simulink model "calibration_model_v2_phase_pid"  (R2015b)
settings: Solver=FixedStepDiscrete  StartTime=0.0  StopTime=inf  FixedStep=.001  RelTol=1e-3
libraries: xpcethercatlib x10, slrtlib x5, simulink x1, dspfdesign x1
settings Model: xpc_rtwmakecfg_data=_xpcethercatlib_  SimulationMode=external  Creator=rtheyyun  LastModifiedBy=tech
settings SolverCC: EnableConcurrentExecution=on  ConcurrentTasks=on
settings DataIOCC: SaveFinalState=on  SaveFormat=StructureWithTime  SignalLoggingSaveFormat=ModelDataLogs  InspectSignalLogs=on
settings OptimizationCC: BlockReduction=off  OptimizeBlockIOStorage=off  BufferReuse=off  GlobalBufferReuse=off  ExpressionFolding=off  ExpressionDepthLimit=2147483647  LocalBlockOutputs=off
settings DebuggingCC: ReadBeforeWriteMsg=DisableAll  WriteAfterWriteMsg=DisableAll  WriteAfterReadMsg=DisableAll  UnderspecifiedInitializationDetection=Classic  MergeDetectMultiDrivingBlocksExec=none  SolverPrmCheckMsg=warning  InheritedTsInSrcMsg=none  FcnCallInpInsideContextMsg=UseLocalSettings  StateNameClashWarn=warning
settings HardwareCC: ProdBitPerPointer=32  ProdLargestAtomicFloat=None  ProdWordSize=32  ProdLongLongMode=on  ProdHWDeviceType=Generic->32-bit x86 compatible
settings RTWCC: SystemTargetFile=slrt.tlc  TemplateMakefile=slrt_default_tmf  Description=Simulink Real-Time  RTWVerbose=off  RTWCompilerOptimization=on
settings SimulinkRealTimeCC: GeneratePreprocessorConditionals=Disable all  xPCisModelTimeout=off  xPCModelTimeoutSecs=20  xPCConcurrentTasks=on
settings ConfigComp: CovModelRefEnable=Off  CovSFcnEnable=off

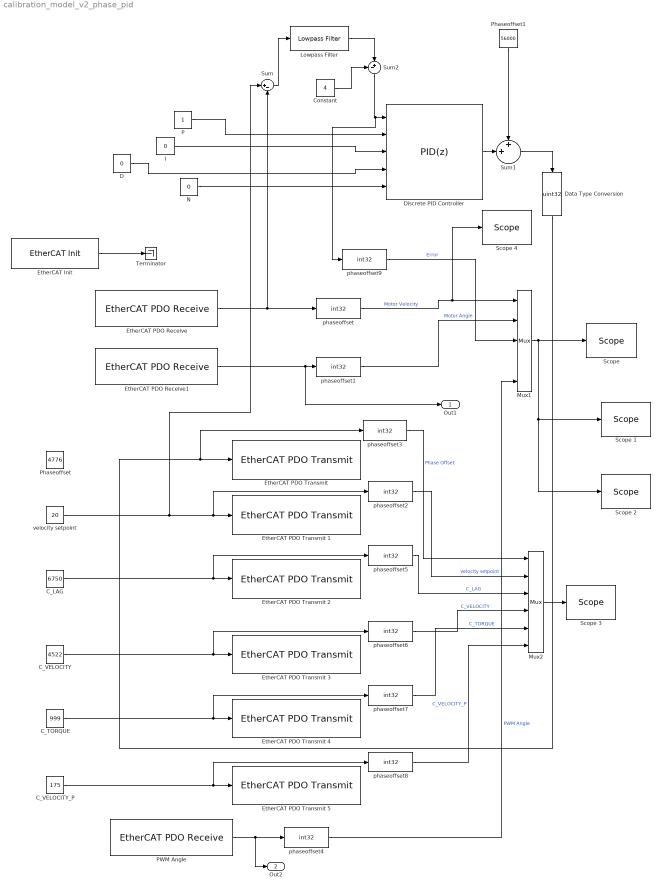
== system calibration_model_v2_phase_pid ==
  C_LAG : Constant  Value=6750  OutDataTypeStr=uint32
  C_TORQUE : Constant  Value=999  OutDataTypeStr=uint32
  C_VELOCITY : Constant  Value=4522  OutDataTypeStr=uint32
  C_VELOCITY_P : Constant  Value=175  OutDataTypeStr=uint32
  Constant : Constant  Value=4
  D : Constant  Value=0
  Data Type Conversion : DataTypeConversion  OutDataTypeStr=uint32
  Discrete PID Controller : simulink/Continuous/PID Controller  Controller=PID  TimeDomain=Discrete-time  SampleTime=-1  IntegratorMethod=Forward Euler  FilterMethod=Forward Euler  Form=Parallel  UseFilter=on  ControllerParametersSource=external  P=1  I=1  D=0  N=100  InitialConditionSource=internal  InitialConditionForIntegrator=0  InitialConditionForFilter=0  ExternalReset=none  LimitOutput=on  UpperSaturationLimit=25536  LowerSaturationLimit=-40000  LinearizeAsGain=off  AntiWindupMode=none  Kb=1  TrackingMode=off  Kt=1  PParamMin=[]  PParamMax=[]  IParamMin=[]  IParamMax=[]  DParamMin=[]  DParamMax=[]  NParamMin=[]  NParamMax=[]  KbParamMin=[]  KbParamMax=[]  KtParamMin=[]  KtParamMax=[]  POutMin=[]  POutMax=[]  IOutMin=[]  IOutMax=[]  DOutMin=[]  DOutMax=[]  NOutMin=[]  NOutMax=[]  KbOutMin=[]  KbOutMax=[]  KtOutMin=[]  KtOutMax=[]  IntegratorOutMin=[]  IntegratorOutMax=[]  FilterOutMin=[]  FilterOutMax=[]  SumOutMin=[]  SumOutMax=[]  SumI1OutMin=[]  SumI1OutMax=[]  SumI2OutMin=[]  SumI2OutMax=[]  SumI3OutMin=[]  SumI3OutMax=[]  SumDOutMin=[]  SumDOutMax=[]  SaturationOutMin=[]  SaturationOutMax=[]  IntegratorContinuousStateAttributes=''  IntegratorStateMustResolveToSignalObject=off  IntegratorRTWStateStorageClass=Auto  FilterContinuousStateAttributes=''  FilterStateMustResolveToSignalObject=off  FilterRTWStateStorageClass=Auto  DifferentiatorICPrevScaledInput=0  DifferentiatorOutMin=[]  DifferentiatorOutMax=[]
  "EtherCAT Init " : xpcethercatlib/EtherCAT Init   Priority=0  config_file=C:\Software\Simulink Realtime\EtherCAT Config files\single_slave_v1.2.xml  device_id=0  pci_bus=2  pci_slot=0  dctuning=2  enaDebug=off  enaDC=off  errLink=on  masterDbg=on  stateChgDbg=on  baseClock=off  masterCfg=on  logFile='c:\dbglog.txt'  sample_time=0.001000
  EtherCAT PDO Receive : xpcethercatlib/EtherCAT PDO Receive  Priority=2  sig_name=Box 1 (FB1111 SPI-Slave).Inputs.motorVelocity  sig_offset=256  sig_type=int16  type_size=16  sig_dim=1  device_id=0  sample_time=0.001000
  EtherCAT PDO Receive1 : xpcethercatlib/EtherCAT PDO Receive  Priority=2  sig_name=Box 1 (FB1111 SPI-Slave).Inputs.motorAngle  sig_offset=240  sig_type=uint16  type_size=16  sig_dim=1  device_id=0  sample_time=0.001000
  "EtherCAT PDO Transmit " : xpcethercatlib/EtherCAT PDO Transmit   Priority=3  sig_name=Box 1 (FB1111 SPI-Slave).Outputs.jointSetpoint  sig_offset=208  sig_type=uint32  type_size=32  sig_dim=1  device_id=0  sample_time=0.001000
  EtherCAT PDO Transmit 1 : xpcethercatlib/EtherCAT PDO Transmit   Priority=3  sig_name=Box 1 (FB1111 SPI-Slave).Outputs.data0  sig_offset=240  sig_type=uint32  type_size=32  sig_dim=1  device_id=0  sample_time=0.001000
  EtherCAT PDO Transmit 2 : xpcethercatlib/EtherCAT PDO Transmit   Priority=3  sig_name=Box 1 (FB1111 SPI-Slave).Outputs.data1  sig_offset=272  sig_type=uint32  type_size=32  sig_dim=1  device_id=0  sample_time=0.001000
  EtherCAT PDO Transmit 3 : xpcethercatlib/EtherCAT PDO Transmit   Priority=3  sig_name=Box 1 (FB1111 SPI-Slave).Outputs.data2  sig_offset=304  sig_type=uint32  type_size=32  sig_dim=1  device_id=0  sample_time=0.001000
  EtherCAT PDO Transmit 4 : xpcethercatlib/EtherCAT PDO Transmit   Priority=3  sig_name=Box 1 (FB1111 SPI-Slave).Outputs.data3  sig_offset=336  sig_type=uint32  type_size=32  sig_dim=1  device_id=0  sample_time=0.001000
  EtherCAT PDO Transmit 5 : xpcethercatlib/EtherCAT PDO Transmit   Priority=3  sig_name=Box 1 (FB1111 SPI-Slave).Outputs.data4  sig_offset=368  sig_type=uint32  type_size=32  sig_dim=1  device_id=0  sample_time=0.001000
  "I " : Constant  Value=0
  Lowpass Filter : dspfdesign/Lowpass Filter  FilterType=FIR  DesignForMinimumOrder=on  FilterOrder=50  PassbandFrequency=10  StopbandFrequency=20  PassbandRipple=0.1  StopbandAttenuation=80  InheritSampleRate=off  SampleRate=1000  roundingMode=Floor  coeffsDataTypeStr=fixdt(1,16)  SimulateUsing=Interpreted execution
  Mux1 : Mux  Inputs=5
  Mux2 : Mux  Inputs=6
  N : Constant  Value=0
  P : Constant
  PWM Angle : xpcethercatlib/EtherCAT PDO Receive  Priority=2  sig_name=Box 1 (FB1111 SPI-Slave).Inputs.jointAngle  sig_offset=208  sig_type=uint32  type_size=32  sig_dim=1  device_id=0  sample_time=0.001000
  Phaseoffset : Constant  Value=4776  OutDataTypeStr=uint32
  Phaseoffset1 : Constant  Value=56000  OutDataTypeStr=uint32
  "Scope " : slrtlib/Displays and Logging/Scope   scopeno=1  scopetype=Target  autostart=on  viewmode=Numerical  formatstr='%15.6f'  grid=on  ylimits=[0,0]  nosamples=3  noprepostsamples=0  interleave=1  triggermode=FreeRun  triggersignal=1  trigsignalfromport=off  triggerlevel=0.0  triggerslope=Either  triggerscope=1  triggersample=0  filename=data.dat  mode=Lazy  writesize=512  autorestart=off  dynamicfilemode=off  maxwritefilesize=512*1024^2
  Scope 1 : slrtlib/Displays and Logging/Scope   scopeno=2  scopetype=Target  autostart=on  viewmode=Graphical sliding  formatstr='%15.6f'  grid=on  ylimits=[0,0]  nosamples=5000  noprepostsamples=0  interleave=1  triggermode=FreeRun  triggersignal=1  trigsignalfromport=off  triggerlevel=0.0  triggerslope=Either  triggerscope=1  triggersample=0  filename=data.dat  mode=Lazy  writesize=512  autorestart=off  dynamicfilemode=off  maxwritefilesize=512*1024^2
  Scope 2 : slrtlib/Displays and Logging/Scope   scopeno=3  scopetype=File  autostart=on  viewmode=Graphical sliding  formatstr='%15.6f'  grid=on  ylimits=[0,0]  nosamples=50000  noprepostsamples=0  interleave=1  triggermode=FreeRun  triggersignal=1  trigsignalfromport=off  triggerlevel=0.0  triggerslope=Either  triggerscope=1  triggersample=0  filename=data.dat  mode=Lazy  writesize=512  autorestart=on  dynamicfilemode=off  maxwritefilesize=512*1024^2
  Scope 3 : slrtlib/Displays and Logging/Scope   scopeno=4  scopetype=Target  autostart=on  viewmode=Numerical  formatstr='%15.6f'  grid=on  ylimits=[0,0]  nosamples=3  noprepostsamples=0  interleave=1  triggermode=FreeRun  triggersignal=1  trigsignalfromport=off  triggerlevel=0.0  triggerslope=Either  triggerscope=1  triggersample=0  filename=data.dat  mode=Lazy  writesize=512  autorestart=off  dynamicfilemode=off  maxwritefilesize=512*1024^2
  Scope 4 : slrtlib/Displays and Logging/Scope   scopeno=5  scopetype=Target  autostart=on  viewmode=Graphical rolling  formatstr='%15.6f'  grid=on  ylimits=[0,0]  nosamples=10000  noprepostsamples=0  interleave=1  triggermode=FreeRun  triggersignal=1  trigsignalfromport=off  triggerlevel=0.0  triggerslope=Either  triggerscope=1  triggersample=0  filename=data.dat  mode=Lazy  writesize=512  autorestart=off  dynamicfilemode=off  maxwritefilesize=512*1024^2
  Sum : Sum  Inputs=|+-
  Sum1 : Sum  Inputs=++|
  Sum2 : Sum  Inputs=-+|
  Terminator : Terminator
  phaseoffset{,1..9} (10 alike) : DataTypeConversion  OutDataTypeStr=int32
  velocity setpoint : Constant  Value=20  OutDataTypeStr=uint32
  Out1 : Outport  OutDataTypeStr=uint16
  Out2 : Outport  Port=2  OutDataTypeStr=uint32
  wires:
  Mux1/1 -> Scope 2/1, Scope 1/1, "Scope "/1
  "EtherCAT Init "/1 -> Terminator/1
  EtherCAT PDO Receive/1 -> phaseoffset/1, Sum/2
  EtherCAT PDO Receive1/1 -> Out1/1, phaseoffset1/1
  phaseoffset1/1 -> Mux1/2  "Motor Angle"
  phaseoffset/1 -> Scope 4/1, Mux1/1  "Motor Velocity"
  phaseoffset3/1 -> Mux2/1  "Phase Offset"
  PWM Angle/1 -> Out2/1, phaseoffset4/1
  phaseoffset4/1 -> Mux1/5  "PWM Angle"
  velocity setpoint/1 -> Sum/1, phaseoffset2/1, EtherCAT PDO Transmit 1/1
  phaseoffset2/1 -> Mux2/2  "velocity setpoint"
  C_LAG/1 -> phaseoffset5/1, EtherCAT PDO Transmit 2/1
  Mux2/1 -> Scope 3/1
  phaseoffset5/1 -> Mux2/3  "C_LAG"
  C_VELOCITY/1 -> phaseoffset6/1, EtherCAT PDO Transmit 3/1
  phaseoffset6/1 -> Mux2/4  "C_VELOCITY"
  C_TORQUE/1 -> phaseoffset7/1, EtherCAT PDO Transmit 4/1
  phaseoffset7/1 -> Mux2/5  "C_TORQUE"
  C_VELOCITY_P/1 -> phaseoffset8/1, EtherCAT PDO Transmit 5/1
  phaseoffset8/1 -> Mux2/6  "C_VELOCITY_P"
  Sum/1 -> Lowpass Filter/1
  Phaseoffset1/1 -> Sum1/1
  Discrete PID Controller/1 -> Sum1/2
  Sum1/1 -> Data Type Conversion/1
  Data Type Conversion/1 -> phaseoffset3/1, "EtherCAT PDO Transmit "/1
  phaseoffset9/1 -> Mux1/3  "Error"
  P/1 -> Discrete PID Controller/2
  "I "/1 -> Discrete PID Controller/3
  D/1 -> Discrete PID Controller/4
  N/1 -> Discrete PID Controller/5
  Lowpass Filter/1 -> Sum2/2
  Sum2/1 -> phaseoffset9/1, Discrete PID Controller/1
  Constant/1 -> Sum2/1
